simulink model "momentumBasedFlying"  (Simulink 9.0)
settings: Solver=FixedStepAuto  StartTime=0.0  StopTime="Config.simulationTime "  FixedStep=Config.Ts  RelTol=1e-3  EnableMultiTasking=on
InitFcn:
  | cd(fileparts(which(bdroot)));
  | initMomentumBasedFlying;
StopFcn:
  | visualizer_demo_idyntree(time.Data,state.Data,Config,desired_x_dx_ddx_dddx_CoM,jetsIntensitiesByWeight);
undefined symbols (not defined in the file or in its folder): Config, config
libraries: WBToolboxLibrary x67, simulink x2
(part 2 of 2)

== matlab function Flying Controller/Dynamics and Kinematics/fromFloatingToCentroidalDynamics/fromState2TandTD ==
  data: M input double; posCoM input double; c_T_b output double; w_H_b input double; posCoMDot input double; basePosDot input double; TDot output double
function [c_T_b, TDot] = centroidalTransformationT_TDot(M, posCoM, w_H_b, posCoMDot, basePosDot)

    [c_T_b, TDot] = centroidalTransformationT_TDot(posCoM, w_H_b(1:3,4), posCoMDot, basePosDot, M);
end
